simulink model "LaneMarkerDetector"  (R2022b)
settings: Solver=FixedStepAuto  StartTime=0.0  StopTime=Inf  RelTol=1e-3  EnableMultiTasking=on
settings Model: Creator=The MathWorks, Inc.  LastModifiedBy=levenT
settings SolverCC: AlgebraicLoopSolver=TrustRegion
settings DataIOCC: SaveOutput=off  SaveTime=off  ReturnWorkspaceOutputs=off
settings OptimizationCC: DefaultParameterBehavior=Inlined  InlineInvariantSignals=on  EnhancedBackFolding=on  PassReuseOutputArgsAs=Individual arguments  ZeroExternalMemoryAtStartup=off  ZeroInternalMemoryAtStartup=off  EfficientFloat2IntCast=on  OptimizeBlockOrder=speed  DifferentSizesBufferReuse=on  OptimizationCustomize=off  EfficientTunableParamExpr=on
settings DebuggingCC: ParameterPrecisionLossMsg=none  ParameterTunabilityLossMsg=error  UnconnectedInputMsg=warning  UnconnectedOutputMsg=warning  UnconnectedLineMsg=warning  BusObjectLabelMismatch=error  PregeneratedLibrarySubsystemCodeDiagnostic=none  SFMachineParentedDataDiag=warning  ArithmeticOperatorsInVariantConditions=warning
settings HardwareCC: ProdLongLongMode=on
settings ModelReferenceCC: EnableRefExpFcnMdlSchedulingChecks=on
settings SFSimCC: SimUseLocalCustomCode=off
settings RTWCC: Description=Embedded Coder  SystemTargetFile=ert.tlc  TemplateMakefile=ert_default_tmf  RTWVerbose=off  RTWUseLocalCustomCode=off  BuildConfiguration=Faster Runs  CodeExecutionProfiling=on  CodeProfilingSaveOptions=AllData  TargetLang=C++  DLArmComputeVersion=19.05
settings CodeAppCC: ForceParamTrailComments=on  IgnoreCustomStorageClasses=off  OperatorAnnotations=on  SimulinkDataObjDesc=on  SFDataObjDesc=on  CustomSymbolStrGlobalVar=$N$M  CustomSymbolStrType=$N$M_T  CustomSymbolStrFcn=APV_$N$M$F  CustomSymbolStrMacro=$N$M  InsertBlockDesc=on
settings ERTTargetCC: TargetLangStandard=C++03 (ISO)  GenerateSampleERTMain=on  CombineSignalStateStructs=on  CodeInterfacePackaging=C++ class  SupportVariableSizeSignals=on  InlinedParameterPlacement=NonHierarchical  RootIOFormat=Structure reference  ERTCustomFileTemplate=example_file_process.tlc
settings ConfigComp: CovScope=ReferencedModels  CovIncludeTopModel=off

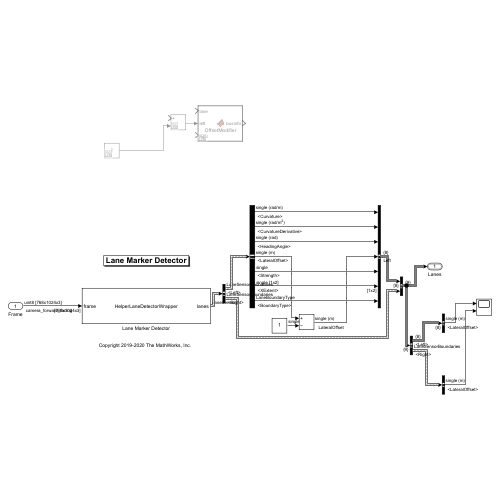
[thumbnail: Simulink's stored preview of the top-level diagram]
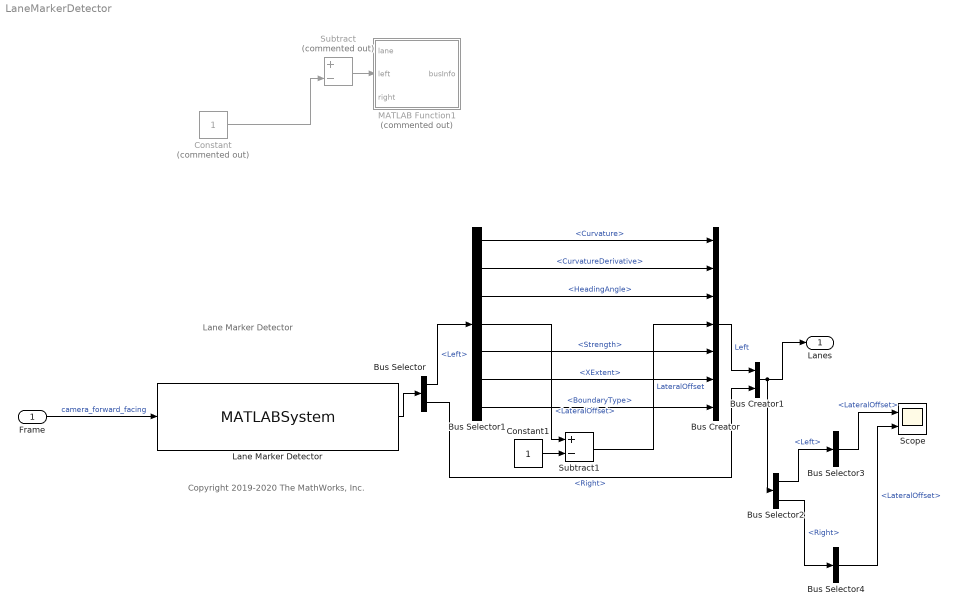
== system LaneMarkerDetector ==
  note: Copyright 2019-2020 The MathWorks, Inc.
  note: Lane Marker Detector
  Frame : Inport  OutDataTypeStr=uint8  PortDimensions=[768 1024 3]  SampleTime=[0.10000000000000001,0]
  Bus Creator : BusCreator  Inputs=7
  Bus Creator1 : BusCreator  Inputs=2
  Bus Selector : BusSelector  OutputSignals=Left,Right
  Bus Selector1 : BusSelector  OutputSignals=Curvature,CurvatureDerivative,HeadingAngle,LateralOffset,Strength,XExtent,BoundaryType
  Bus Selector2 : BusSelector  OutputSignals=Left,Right
  Bus Selector3 : BusSelector  OutputSignals=LateralOffset
  Bus Selector4 : BusSelector  OutputSignals=LateralOffset
  Constant : Constant  Commented=on
  Constant1 : Constant  OutDataTypeStr=single
  Lane Marker Detector : MATLABSystem  System=HelperLaneDetectorWrapper  EnableLaneTracker=on  EnableDisplays=on  Camera=camera  SimulateUsing=Interpreted execution
      mask Type: HelperLaneDetectorWrapper
      mask Display:
      | disp('HelperLaneDetectorWrapper');
      | port_label('input',1,'frame');
      | port_label('output',1,'lanes');
  MATLAB Function1 : MATLAB Function  Commented=on  TreatAsAtomicUnit=on
  Scope : Scope  NumInputPorts=2
  Subtract : Sum  Commented=on  Inputs=+-
  Subtract1 : Sum  Inputs=+-
  Lanes : Outport  OutDataTypeStr=Bus: LaneSensor  PortDimensions=[1 1]  SampleTime=[0.10000000000000001,0]  BusOutputAsStruct=on
  wires:
  Frame/1 -> Lane Marker Detector/1  "camera_forward_facing"
  Constant/1 -> Subtract/2
  Subtract/1 -> MATLAB Function1/2(left)
  Lane Marker Detector/1 -> Bus Selector/1
  Bus Selector/1 -> Bus Selector1/1  "<Left>"
  Bus Selector1/1 -> Bus Creator/1  "<Curvature>"
  Bus Selector1/2 -> Bus Creator/2  "<CurvatureDerivative>"
  Bus Selector1/3 -> Bus Creator/3  "<HeadingAngle>"
  Bus Selector1/5 -> Bus Creator/5  "<Strength>"
  Bus Selector1/6 -> Bus Creator/6  "<XExtent>"
  Bus Selector1/7 -> Bus Creator/7  "<BoundaryType>"
  Constant1/1 -> Subtract1/2
  Bus Creator/1 -> Bus Creator1/1  "Left"
  Bus Selector/2 -> Bus Creator1/2  "<Right>"
  Bus Creator1/1 -> Bus Selector2/1, Lanes/1
  Bus Selector1/4 -> Subtract1/1  "<LateralOffset>"
  Subtract1/1 -> Bus Creator/4  "LateralOffset"
  Bus Selector2/1 -> Bus Selector3/1  "<Left>"
  Bus Selector2/2 -> Bus Selector4/1  "<Right>"
  Bus Selector3/1 -> Scope/1  "<LateralOffset>"
  Bus Selector4/1 -> Scope/2  "<LateralOffset>"

== matlab function LaneMarkerDetector/MATLAB Function1 ==
  data: lane input; busInfo output; left input; right input
function busInfo = OffsetModifier(lane,left,right)

newlane = lane;
newlane.Left.LateralOffset = left;
newlane.Right.LateralOffset= right;

busInfo = Simulink.Bus.createObject(newlane);
